simulink model "Simulink_Respuesta_Escalon_sin_Perturbacion"  (R2020b)
settings: Solver=VariableStepAuto  StartTime=0.0  StopTime=2  RelTol=1e-3
values from neighbouring files (symbols this model uses):
  Amplitud_referencia = 1    [Contolador_Por_Modelo_Interno.m]
  KM = 1    [Contolador_Por_Modelo_Interno.m]
  TaoF = TaoM/2    (= 0.025)    [Contolador_Por_Modelo_Interno.m]
  TaoM = 0.05    [Contolador_Por_Modelo_Interno.m]
  Tiempo_escalon = 0.5    [Contolador_Por_Modelo_Interno.m]
  TL = 0.1    [Contolador_Por_Modelo_Interno.m]
settings Model: Creator=Fernando Madera  LastModifiedBy=Fernando Madera

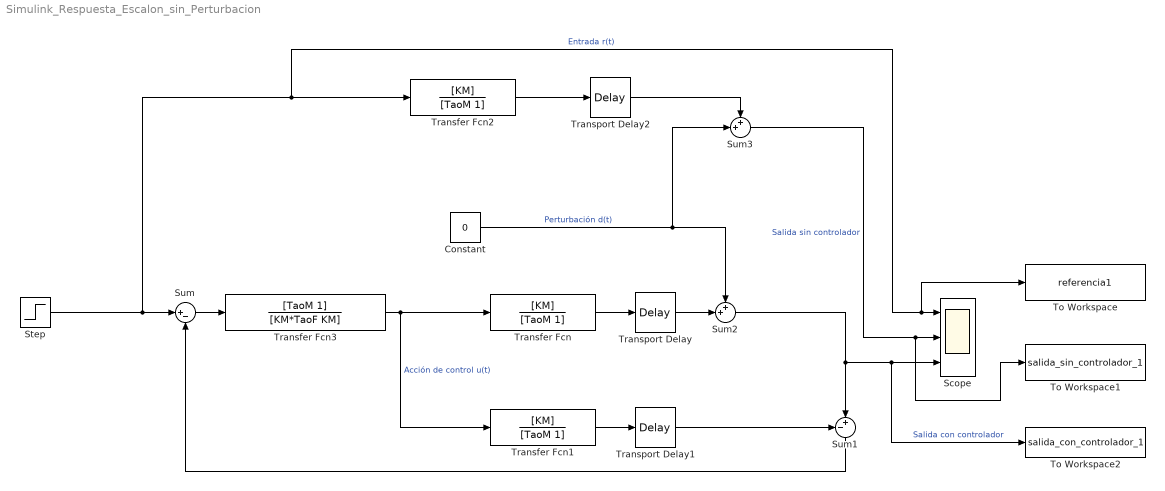
== system Simulink_Respuesta_Escalon_sin_Perturbacion ==
  Constant : Constant  Value=0
  Scope : Scope  NumInputPorts=3
  Step : Step  Time=Tiempo_escalon  After=Amplitud_referencia  SampleTime=0
  Sum : Sum  Inputs=|+-
  Sum1 : Sum  Inputs=-+|
  Sum2 : Sum  Inputs=++|
  Sum3 : Sum  Inputs=++|
  To Workspace : ToWorkspace  VariableName=referencia1  SaveFormat=Timeseries  SampleTime=-1
  To Workspace1 : ToWorkspace  VariableName=salida_sin_controlador_1  SaveFormat=Timeseries  SampleTime=-1
  To Workspace2 : ToWorkspace  VariableName=salida_con_controlador_1  SaveFormat=Timeseries  SampleTime=-1
  Transfer Fcn : TransferFcn  Numerator=[KM]  Denominator=[TaoM 1]
  Transfer Fcn1 : TransferFcn  Numerator=[KM]  Denominator=[TaoM 1]
  Transfer Fcn2 : TransferFcn  Numerator=[KM]  Denominator=[TaoM 1]
  Transfer Fcn3 : TransferFcn  Numerator=[TaoM 1]  Denominator=[KM*TaoF KM]
  Transport Delay : TransportDelay  DelayTime=TL
  Transport Delay1 : TransportDelay  DelayTime=TL
  Transport Delay2 : TransportDelay  DelayTime=TL
  wires:
  Transport Delay/1 -> Sum2/2
  Transfer Fcn/1 -> Transport Delay/1
  Transport Delay2/1 -> Sum3/1
  Step/1 -> To Workspace/1, Scope/1, Transfer Fcn2/1, Sum/1  "Entrada r(t)"
  Transport Delay1/1 -> Sum1/1
  Sum1/1 -> Sum/2
  Sum/1 -> Transfer Fcn3/1
  Sum2/1 -> To Workspace2/1, Scope/3, Sum1/2  "Salida con controlador"
  Transfer Fcn3/1 -> Transfer Fcn/1, Transfer Fcn1/1  "Acción de control u(t)"
  Constant/1 -> Sum3/2, Sum2/1  "Perturbación d(t)"
  Transfer Fcn1/1 -> Transport Delay1/1
  Transfer Fcn2/1 -> Transport Delay2/1
  Sum3/1 -> To Workspace1/1, Scope/2  "Salida sin controlador"
